simulink model "APP"  (R2022b)
settings: Solver=FixedStepAuto  StartTime=0.0  StopTime=10.0  RelTol=1e-3
settings Model: Creator=MAAM  LastModifiedBy=MAAM
settings OptimizationCC: DefaultParameterBehavior=Inlined  UseDivisionForNetSlopeComputation=on  GainParamInheritBuiltInType=on  UseFloatMulNetSlope=on  InlineInvariantSignals=on  PassReuseOutputArgsAs=Individual arguments  ZeroExternalMemoryAtStartup=off  ZeroInternalMemoryAtStartup=off  NoFixptDivByZeroProtection=on  EfficientFloat2IntCast=on  LifeSpan=1  OptimizeBlockOrder=speed  DifferentSizesBufferReuse=on  EfficientTunableParamExpr=on
settings DebuggingCC: ParameterTunabilityLossMsg=error
settings HardwareCC: ProdLongLongMode=on
settings SFSimCC: MATLABDynamicMemAlloc=off
settings RTWCC: Description=Embedded Coder  SystemTargetFile=ert.tlc  TemplateMakefile=ert_default_tmf  CreateSILPILBlock=SIL
settings CodeAppCC: ForceParamTrailComments=on  IgnoreCustomStorageClasses=off  OperatorAnnotations=on  SimulinkDataObjDesc=on  SFDataObjDesc=on  CustomSymbolStrGlobalVar=rt$N$M  CustomSymbolStrType=$N$M  CustomSymbolStrFcn=$N$M$F  CustomSymbolStrMacro=$N$M  InsertBlockDesc=on
settings ERTTargetCC: TargetLangStandard=C99 (ISO)  GenerateSampleERTMain=on  IncludeMdlTerminateFcn=off  CombineSignalStateStructs=on  SupportAbsoluteTime=off  SupportComplex=off  SupportNonInlinedSFcns=on  InlinedParameterPlacement=NonHierarchical  ERTCustomFileTemplate=example_file_process.tlc  ERTFilePackagingFormat=CompactWithDataFile

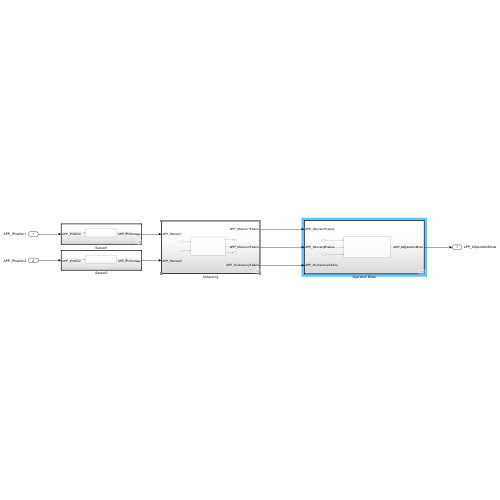
[thumbnail: Simulink's stored preview of the top-level diagram]
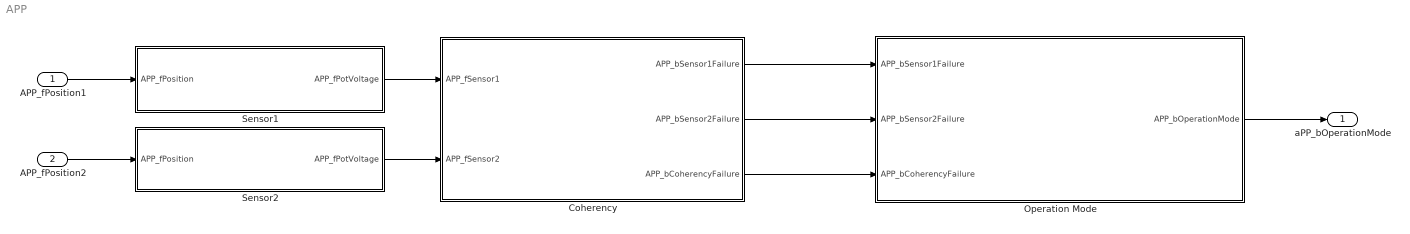
== system APP ==
  APP_fPosition1 : Inport  OutDataTypeStr=single
  APP_fPosition2 : Inport  Port=2  OutDataTypeStr=single
  Coherency : Subsystem  TreatAsAtomicUnit=on
  Operation Mode : Subsystem  TreatAsAtomicUnit=on
  Sensor1 : Subsystem  TreatAsAtomicUnit=on
  Sensor2 : Subsystem  TreatAsAtomicUnit=on
  aPP_bOperationMode : Outport
  wires:
  Coherency/1(APP_bSensor1Failure) -> Operation Mode/1(APP_bSensor1Failure)
  Coherency/2(APP_bSensor2Failure) -> Operation Mode/2(APP_bSensor2Failure)
  Coherency/3(APP_bCoherencyFailure) -> Operation Mode/3(APP_bCoherencyFailure)
  Operation Mode/1(APP_bOperationMode) -> aPP_bOperationMode/1
  APP_fPosition1/1 -> Sensor1/1(APP_fPosition)
  Sensor1/1(APP_fPotVoltage) -> Coherency/1(APP_fSensor1)
  APP_fPosition2/1 -> Sensor2/1(APP_fPosition)
  Sensor2/1(APP_fPotVoltage) -> Coherency/2(APP_fSensor2)

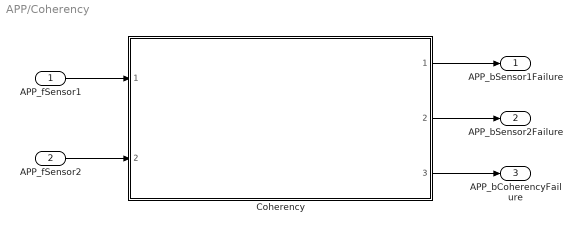
== system APP/Coherency ==
  APP_fSensor1 : Inport  OutDataTypeStr=single
  APP_fSensor2 : Inport  Port=2  OutDataTypeStr=single
  Coherency : Subsystem  TreatAsAtomicUnit=on  ReferencedSubsystem=APPC  Max=4.5  Min=0.5
  APP_bSensor1Failure : Outport  OutDataTypeStr=boolean
  APP_bSensor2Failure : Outport  Port=2  OutDataTypeStr=boolean
  APP_bCoherencyFailure : Outport  Port=3  OutDataTypeStr=boolean
  wires:
  Coherency/3 -> APP_bCoherencyFailure/1
  Coherency/2 -> APP_bSensor2Failure/1
  Coherency/1 -> APP_bSensor1Failure/1
  APP_fSensor1/1 -> Coherency/1
  APP_fSensor2/1 -> Coherency/2

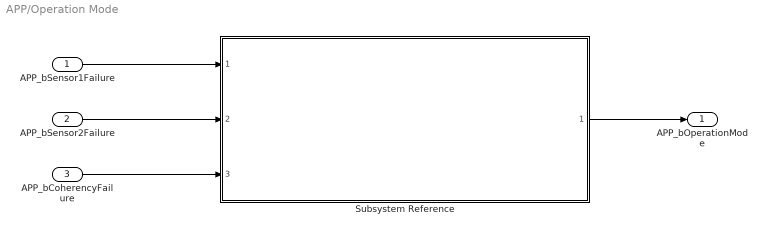
== system APP/Operation Mode ==
  APP_bSensor1Failure : Inport
  APP_bSensor2Failure : Inport  Port=2
  APP_bCoherencyFailure : Inport  Port=3
  Subsystem Reference : Subsystem  ReferencedSubsystem=APPM
  APP_bOperationMode : Outport
  wires:
  Subsystem Reference/1 -> APP_bOperationMode/1
  APP_bSensor1Failure/1 -> Subsystem Reference/1
  APP_bSensor2Failure/1 -> Subsystem Reference/2
  APP_bCoherencyFailure/1 -> Subsystem Reference/3

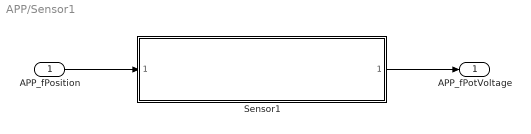
== system APP/Sensor1 ==
  APP_fPosition : Inport
  Sensor1 : Subsystem  TreatAsAtomicUnit=on  ReferencedSubsystem=APPS  Max=4.5  Min=0.5
  APP_fPotVoltage : Outport
  wires:
  Sensor1/1 -> APP_fPotVoltage/1
  APP_fPosition/1 -> Sensor1/1

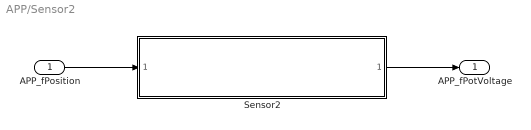
== system APP/Sensor2 ==
  APP_fPosition : Inport
  Sensor2 : Subsystem  TreatAsAtomicUnit=on  ReferencedSubsystem=APPS  Max=0.5  Min=4.5
  APP_fPotVoltage : Outport
  wires:
  Sensor2/1 -> APP_fPotVoltage/1
  APP_fPosition/1 -> Sensor2/1
